simulink model "Simulacao_Continua"  (R2013b)
settings: Solver=ode45  StartTime=0.0  StopTime=5  RelTol=1e-3
values from neighbouring files (symbols this model uses):
  A = Ap    [Main.m]
  B = Bp    [Main.m]
  C = Cp    [Main.m]
  D = Dp    [Main.m]
  dt = 0.1    [Main.m]
  Ka = -0.04238    [Main.m]
  Ki = 0.8426    [Main.m]
  Kq = -0.4098    [Main.m]
settings Model: Creator=Eduardo  LastModifiedBy=Eduardo

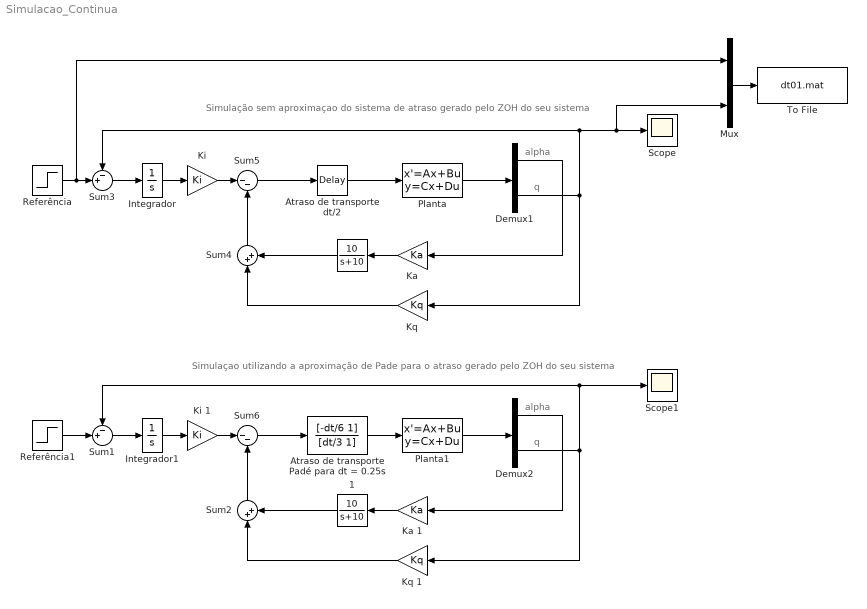
== system Simulacao_Continua ==
  note: Simulaçao utilizando a aproximação de Pade para o atraso gerado pelo ZOH do seu sistema
  note: Simulação sem aproximaçao do sistema de atraso gerado pelo ZOH do seu sistema
  note: alpha
  note: q
  note: alpha
  note: q
  "   " : TransferFcn  Numerator=[10]  Denominator=[1 10]
  "   1" : TransferFcn  Numerator=[10]  Denominator=[1 10]
  "   Atraso de transporte Padé para dt = 0.25s " : TransferFcn  Numerator=[-dt/6 1]  Denominator=[dt/3 1]
  Atraso de transporte dt/2 : TransportDelay  DelayTime=dt/2
  Demux1 : Demux  Outputs=2
  Demux2 : Demux  Outputs=2
  Integrador : TransferFcn  Denominator=[1 0]
  Integrador1 : TransferFcn  Denominator=[1 0]
  "Ka " : Gain  Gain=Ka
  Ka 1 : Gain  Gain=Ka
  "Ki " : Gain  Gain=Ki
  Ki 1 : Gain  Gain=Ki
  "Kq " : Gain  Gain=Kq
  Kq 1 : Gain  Gain=Kq
  Mux : Mux  Inputs=2
  Planta : StateSpace  A=A  B=B  C=C  D=D  X0=0
  Planta1 : StateSpace  A=A  B=B  C=C  D=D  X0=0
  Referência : Step  SampleTime=0
  Referência1 : Step  SampleTime=0
  Scope : Scope
  Scope1 : Scope
  Sum1 : Sum  Inputs=-+|
  Sum2 : Sum  Inputs=|++
  Sum3 : Sum  Inputs=-+|
  Sum4 : Sum  Inputs=|++
  Sum5 : Sum  Inputs=|--
  Sum6 : Sum  Inputs=|--
  To File : ToFile  Filename=dt01.mat  SaveFormat=Timeseries
  wires:
  Integrador/1 -> "Ki "/1
  "Ka "/1 -> "   "/1
  "Kq "/1 -> Sum4/1
  "   "/1 -> Sum4/2
  "Ki "/1 -> Sum5/1
  Sum4/1 -> Sum5/2
  Referência/1 -> Mux/1, Sum3/2
  Sum3/1 -> Integrador/1
  Demux1/2 -> "Kq "/1, Scope/1, Mux/2, Sum3/1
  Demux1/1 -> "Ka "/1
  Planta/1 -> Demux1/1
  Sum5/1 -> Atraso de transporte dt/2/1
  Atraso de transporte dt/2/1 -> Planta/1
  Integrador1/1 -> Ki 1/1
  Ka 1/1 -> "   1"/1
  Kq 1/1 -> Sum2/1
  "   1"/1 -> Sum2/2
  Ki 1/1 -> Sum6/1
  Sum2/1 -> Sum6/2
  Referência1/1 -> Sum1/2
  Sum1/1 -> Integrador1/1
  Demux2/2 -> Kq 1/1, Scope1/1, Sum1/1
  Demux2/1 -> Ka 1/1
  Planta1/1 -> Demux2/1
  Sum6/1 -> "   Atraso de transporte Padé para dt = 0.25s "/1
  "   Atraso de transporte Padé para dt = 0.25s "/1 -> Planta1/1
  Mux/1 -> To File/1
